simulink model "Diode_Rectifier_Three_Phase_RLload"  (R2018b)
settings: Solver=VariableStepAuto  StartTime=0.0  StopTime=0.1  RelTol=1e-3
libraries: powerlib x21
settings Model: Creator=A.hey  LastModifiedBy=A.hey

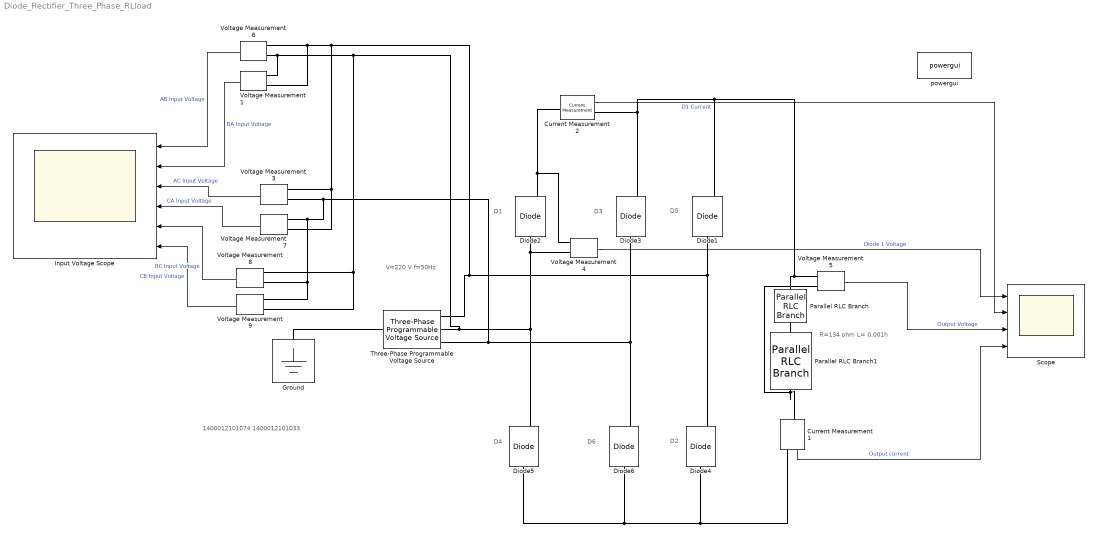
== system Diode_Rectifier_Three_Phase_RLload ==
  note: R=134 ohm
      | L= 0.001h
  note: 1400012101074
      | 1400012101033
  note: D1
  note: V=220 V
      | f=50Hz
  note: D3
  note: D5
  note: D4
  note: D6
  note: D2
  " Scope " : Scope  NumInputPorts=4
  Current Measurement1 : powerlib/Measurements/Current Measurement  PhasorSimulation=off  OutputType=Complex  PSBequivalent=0
  Current Measurement2 : powerlib/Measurements/Current Measurement  PhasorSimulation=off  OutputType=Complex  PSBequivalent=0
  Diode{1..6} (6 alike) : powerlib/Power Electronics/Diode  Ron=0.001  Lon=0  Vf=0.8  IC=0  UseSnubber=0  Rs=500  Cs=250e-9  Measurements=on
  Ground : powerlib/Elements/Ground  LConnTagsString=a
  "Input Voltage Scope " : Scope  NumInputPorts=6
  Parallel RLC Branch : powerlib/Elements/Parallel RLC Branch  LConnTagsString=a  RConnTagsString=__new0  BranchType=R  Resistance=134  Inductance=1e-3  SetiL0=off  InitialCurrent=0  Capacitance=1e-6  Setx0=off  InitialVoltage=0  Measurements=None
  Parallel RLC Branch1 : powerlib/Elements/Parallel RLC Branch  LConnTagsString=a  RConnTagsString=__new0  BranchType=L  Resistance=134  Inductance=1e-3  SetiL0=off  InitialCurrent=0  Capacitance=1e-6  Setx0=off  InitialVoltage=0  Measurements=None
  Three-Phase Programmable Voltage Source : powerlib/Electrical Sources/Three-Phase Programmable Voltage Source  PositiveSequence="[220  0 50]"  VariationEntity=None  VariationType=Table of time-amplitude pairs  VariationTypeAlt=Step  VariationStep=0.5  VariationRate=10  VariationMagnitude=0.3  VariationFrequency=2  VariationTiming=[1 2]  VariationPhaseA=off  Amplitudes=[1 0.8 1.2 1.0]  TimeValues=[0 0.1 0.15 0.2]  HarmonicGeneration=off  HarmonicA=[3 0.2 -25 0]  HarmonicB=[2 0.15 35 2]  Timing="[0.05  3]"  BusType=swing  Pref=0  Qref=0  Qmin=-inf  Qmax=inf
  Voltage Measurement{1,3..9} (8 alike) : powerlib/Measurements/Voltage Measurement  PhasorSimulation=off  OutputType=Complex  PSBequivalent=0
  powergui : powerlib/powergui  Priority=1  SimulationMode=Continuous  SampleTime=50e-6  frequency=60  Iterations=50  frequencyindice=50  Pbase=100e6  ErrMax=1e-4  UnitsV=kV  UnitsW=MW  buscounter=0  FunctionMessages=off  echomessages=off  EnableUseOfTLC=off  CurrentSourceSwitches=off  DisableSnubberDevices=off  DisableRonSwitches=off  DisableVfSwitches=off  DisplayEquations=off  SolverType=Tustin/Backward Euler (TBE)  Interpol=off  ExternalGateDelay=off  methode=off  Ts=100  x0status=blocks  SPID=on  SwTol=0  HookPort=off  RestoreLinks=warning  ResistiveCurrentMeasurement=off  Frange=[0:2:500]  Ylog=off  Xlog=on  ShowGrid=off  save=off  variable=ZData  structure=0  ZoomFFT=off  StartTime=0.0  cycles=1  DisplayStyle=1  fundamental=60  FreqAxis=off  MaxFrequency=1000  frequencyindicesteady=1  RmsSteady=1  display=off
  wires:
  Voltage Measurement5/1 -> " Scope "/3  "Output Voltage"
  Current Measurement1/1 -> " Scope "/4  "Output current"
  Voltage Measurement4/1 -> " Scope "/1  "Diode 1 Voltage"
  Current Measurement2/1 -> " Scope "/2  "D1 Current"
  Voltage Measurement1/1 -> "Input Voltage Scope "/2  "BA Input Voltage"
  Voltage Measurement8/1 -> "Input Voltage Scope "/5  "BC Input Voltage"
  Voltage Measurement3/1 -> "Input Voltage Scope "/3  "AC Input Voltage"
  Voltage Measurement6/1 -> "Input Voltage Scope "/1  "AB Input Voltage"
  Voltage Measurement9/1 -> "Input Voltage Scope "/6  "CB Input Voltage"
  Voltage Measurement7/1 -> "Input Voltage Scope "/4  "CA Input Voltage"
  connections:
  Voltage Measurement7/LConn1 -- Voltage Measurement9/LConn1 -- Voltage Measurement8/LConn2 -- Diode6/RConn1 -- Diode3/LConn1 -- Three-Phase Programmable Voltage Source/RConn3 -- Voltage Measurement3/LConn2
  Voltage Measurement8/LConn1 -- Voltage Measurement9/LConn2 -- Diode5/RConn1 -- Voltage Measurement4/LConn1 -- Diode2/LConn1 -- Three-Phase Programmable Voltage Source/RConn2 -- Voltage Measurement1/LConn1 -- Voltage Measurement6/LConn2
  Parallel RLC Branch/RConn1 -- Parallel RLC Branch1/LConn1
  Parallel RLC Branch/LConn1 -- Diode1/RConn1 -- Current Measurement2/RConn1 -- Diode3/RConn1 -- Voltage Measurement5/LConn1
  Ground/LConn1 -- Three-Phase Programmable Voltage Source/LConn1
  Diode2/RConn1 -- Voltage Measurement4/LConn2 -- Current Measurement2/LConn1
  Diode6/LConn1 -- Diode5/LConn1 -- Current Measurement1/RConn1 -- Diode4/LConn1
  Parallel RLC Branch1/RConn1 -- Current Measurement1/LConn1 -- Voltage Measurement5/LConn2
  Diode4/RConn1 -- Three-Phase Programmable Voltage Source/RConn1 -- Voltage Measurement7/LConn2 -- Voltage Measurement3/LConn1 -- Voltage Measurement1/LConn2 -- Voltage Measurement6/LConn1 -- Diode1/LConn1
